simulink model "teste_1"  (R2018a)
settings: Solver=VariableStepAuto  StartTime=0.0  StopTime=10.0  RelTol=1e-3
libraries: simulink x1
settings Model: Creator=juan-  LastModifiedBy=juan-

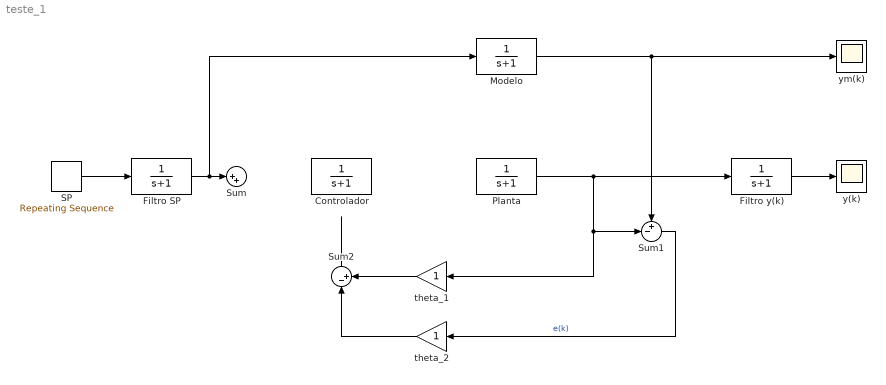
== system teste_1 ==
  Controlador : TransferFcn  Denominator=[1 1]
  Filtro SP : TransferFcn  Denominator=[1 1]
  Filtro y(k) : TransferFcn  Denominator=[1 1]
  "Modelo " : TransferFcn  Denominator=[1 1]
  Planta : TransferFcn  Denominator=[1 1]
  SP : simulink/Sources/Repeating Sequence  rep_seq_t=[0 2]  rep_seq_y=[0 2]
  Sum : Sum  Inputs=|++
  Sum1 : Sum  Inputs=+-|
  Sum2 : Sum  Inputs=|-+
  theta_1 : Gain
  theta_2 : Gain
  y(k) : Scope
  ym(k) : Scope
  wires:
  Filtro y(k)/1 -> y(k)/1
  SP/1 -> Filtro SP/1
  Planta/1 -> theta_1/1, Sum1/2, Filtro y(k)/1
  Filtro SP/1 -> "Modelo "/1, Sum/1
  "Modelo "/1 -> ym(k)/1, Sum1/1
  theta_1/1 -> Sum2/2
  Sum1/1 -> theta_2/1  "e(k)"
  theta_2/1 -> Sum2/1
  Sum2/1 -> ?
